simulink library "ValveCmdLib"  (R2026a)
settings: Solver=VariableStepAuto
Description:
  | Copyright 2022-2026 The MathWorks, Inc.
settings Model: Creator=gabri  LastModifiedBy=smiller

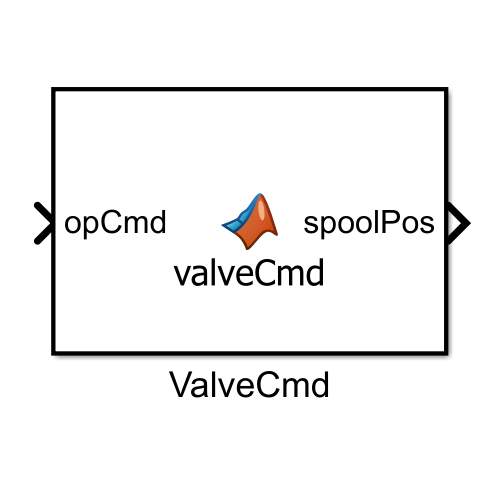
[thumbnail: Simulink's stored preview of the top-level diagram]
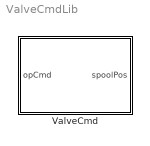
== system ValveCmdLib ==
  ValveCmd : MATLAB Function  TreatAsAtomicUnit=on

== matlab function ValveCmdLib/ValveCmd ==
  data: opCmd input; spoolPos output
function spoolPos  = valveCmd(opCmd)
% Local constants
fullOpenMinCmd = 0.2;

% Initialize outputs
spoolPos = 0;

% Determine spool position
if opCmd >= fullOpenMinCmd
    spoolPos = 5;
elseif opCmd <= -1*fullOpenMinCmd
    spoolPos = -5;
elseif opCmd > 0
    spoolPos = interp1([0 fullOpenMinCmd],[0 5],opCmd);
elseif opCmd < 0
    spoolPos = interp1([-1*fullOpenMinCmd 0],[-5 0],opCmd);
end
